simulink library "mbrt_lib_level1"  (R2023b)
settings: Solver=VariableStepAuto  StartTime=0.0  StopTime=10.0  RelTol=1e-3
values from neighbouring files (symbols this model uses):
  P_cpid_BehaviorPublish = uint64(12)    [i01_data.m]
  P_cpid_CameraStart = uint64(1)    [i01_data.m]
undefined symbols (not defined in the file or in its folder): cpseq, cpseq_SL_Info, cur_cpid, health, seqctr, time
libraries: ros2lib x4, mbrt_lib_level0 x2
settings Model: Creator=ftraenkle  LastModifiedBy=ftraenkle
settings SolverCC: AlgebraicLoopSolver=TrustRegion
settings OptimizationCC: ReuseModelBlockBuffer=off
settings DebuggingCC: UnconnectedInputMsg=warning  UnconnectedOutputMsg=warning  UnconnectedLineMsg=warning
settings ModelReferenceCC: EnableRefExpFcnMdlSchedulingChecks=on
settings RTWCC: DLArmComputeVersion=19.05

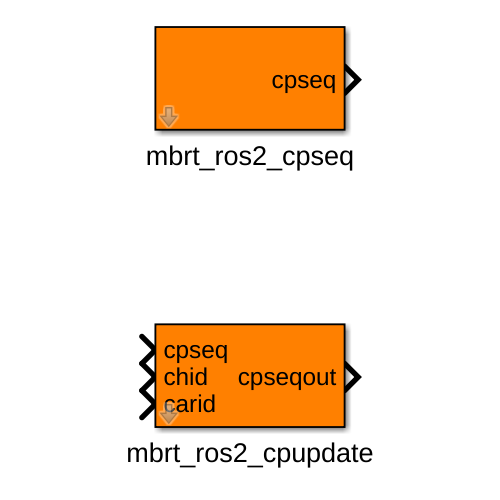
[thumbnail: Simulink's stored preview of the top-level diagram]
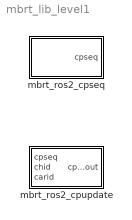
== system mbrt_lib_level1 ==
  mbrt_ros2_cpseq : Subsystem  mask{P_cur_cpid=P_cpid_CameraStart}
      mask prompts: P_cur_cpid "Current Checkpoint Id"
  mbrt_ros2_cpupdate : Subsystem  mask{P_cur_cpid=P_cpid_BehaviorPublish}
      mask prompts: P_cur_cpid "Current Checkpoint Id"

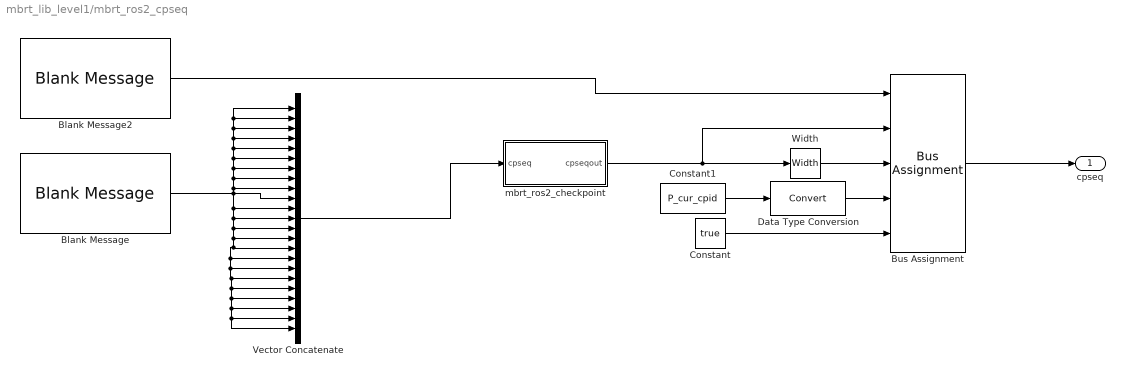
== system mbrt_lib_level1/mbrt_ros2_cpseq ==
  Blank Message : ros2lib/Blank Message  messageClass=Message  entityType=mbsafemsgs/Checkpoint  messageType=mbsafemsgs/Checkpoint  SampleTime=inf
  Blank Message2 : ros2lib/Blank Message  messageClass=Message  entityType=mbsafemsgs/CheckpointSequence  messageType=mbsafemsgs/CheckpointSequence  SampleTime=inf
  Bus Assignment : BusAssignment  AssignedSignals=cpseq,cpseq_SL_Info.CurrentLength,cur_cpid,health
  Constant : Constant  Value=true  OutDataTypeStr=boolean
  Constant1 : Constant  Value=P_cur_cpid
  Data Type Conversion : DataTypeConversion  SaturateOnIntegerOverflow=off  RndMeth=Floor
  Vector Concatenate : Concatenate  NumInputs=P_cp_cnt
  Width : Width  DataType=uint32
  mbrt_ros2_checkpoint : Subsystem
  cpseq : Outport
  wires:
  mbrt_ros2_checkpoint/1(cpseqout) -> Width/1, Bus Assignment/2
  Blank Message2/1 -> Bus Assignment/1
  Data Type Conversion/1 -> Bus Assignment/4
  Blank Message/1 -> Vector Concatenate/8, Vector Concatenate/7, Vector Concatenate/6, Vector Concatenate/5, Vector Concatenate/1, Vector Concatenate/2, Vector Concatenate/3, Vector Concatenate/4, Vector Concatenate/9, Vector Concatenate/10, Vector Concatenate/11, Vector Concatenate/12, Vector Concatenate/13, Vector Concatenate/14, Vector Concatenate/15, Vector Concatenate/17, Vector Concatenate/18, Vector Concatenate/19, Vector Concatenate/20, Vector Concatenate/21, Vector Concatenate/23, Vector Concatenate/22, Vector Concatenate/16
  Vector Concatenate/1 -> mbrt_ros2_checkpoint/1(cpseq)
  Width/1 -> Bus Assignment/3
  Bus Assignment/1 -> cpseq/1
  Constant1/1 -> Data Type Conversion/1
  Constant/1 -> Bus Assignment/5

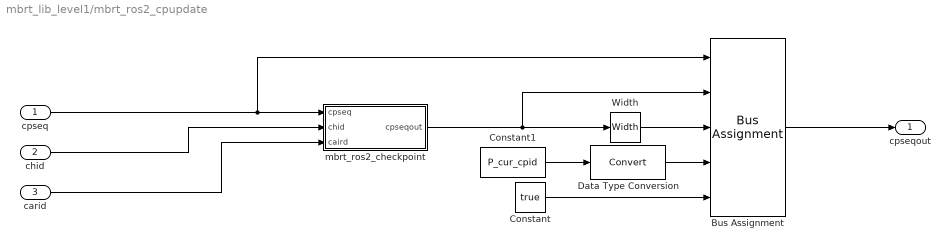
== system mbrt_lib_level1/mbrt_ros2_cpupdate ==
  cpseq : Inport
  chid : Inport  Port=2
  carid : Inport  Port=3
  Bus Assignment : BusAssignment  AssignedSignals=cpseq,cpseq_SL_Info.CurrentLength,cur_cpid,health
  Constant : Constant  Value=true  OutDataTypeStr=boolean
  Constant1 : Constant  Value=P_cur_cpid
  Data Type Conversion : DataTypeConversion  SaturateOnIntegerOverflow=off  RndMeth=Floor
  Width : Width  DataType=uint32
  mbrt_ros2_checkpoint : Subsystem
  cpseqout : Outport
  wires:
  carid/1 -> mbrt_ros2_checkpoint/3(caird)
  chid/1 -> mbrt_ros2_checkpoint/2(chid)
  Bus Assignment/1 -> cpseqout/1
  mbrt_ros2_checkpoint/1(cpseqout) -> Width/1, Bus Assignment/2
  Data Type Conversion/1 -> Bus Assignment/4
  Width/1 -> Bus Assignment/3
  cpseq/1 -> mbrt_ros2_checkpoint/1(cpseq), Bus Assignment/1
  Constant1/1 -> Data Type Conversion/1
  Constant/1 -> Bus Assignment/5

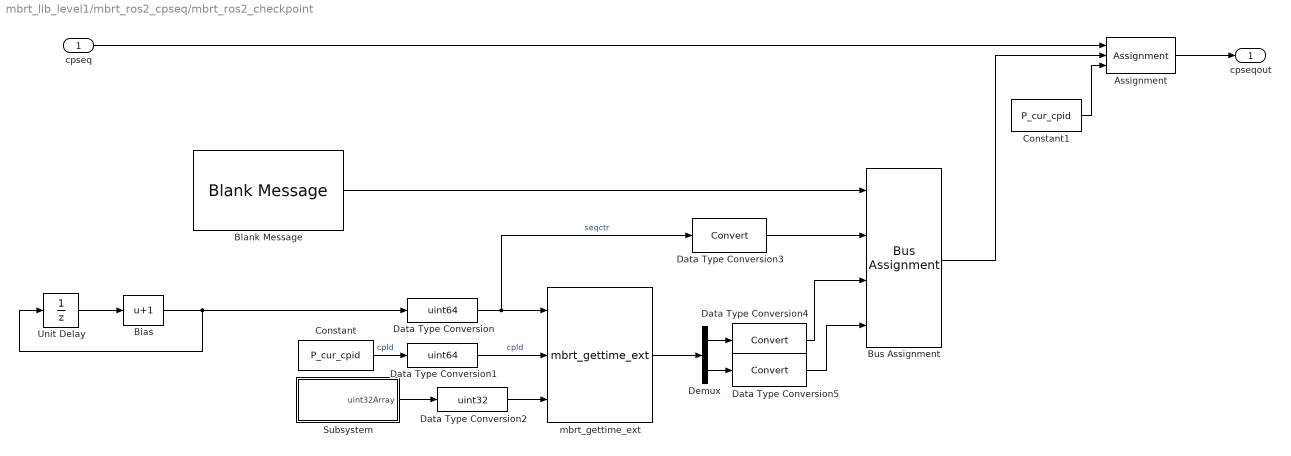
== system mbrt_lib_level1/mbrt_ros2_cpseq/mbrt_ros2_checkpoint ==
  cpseq : Inport
  Assignment : Assignment  IndexMode=Zero-based  DiagnosticForDimensions=Warning  IndexOptions=Index vector (port)  Indices=[1]  OutputSizes=1
  Bias : Bias  Bias=1  SaturateOnIntegerOverflow=off
  Blank Message : ros2lib/Blank Message  messageClass=Message  entityType=mbsafemsgs/Checkpoint  messageType=mbsafemsgs/Checkpoint  SampleTime=inf
  Bus Assignment : BusAssignment  AssignedSignals=seqctr,time.sec,time.nanosec
  Constant : Constant  Value=P_cur_cpid
  Constant1 : Constant  Value=P_cur_cpid
  Data Type Conversion : DataTypeConversion  OutDataTypeStr=uint64  SaturateOnIntegerOverflow=off  RndMeth=Floor
  Data Type Conversion1 : DataTypeConversion  OutDataTypeStr=uint64  SaturateOnIntegerOverflow=off  RndMeth=Floor
  Data Type Conversion2 : DataTypeConversion  OutDataTypeStr=uint32  SaturateOnIntegerOverflow=off  RndMeth=Floor
  Data Type Conversion3 : DataTypeConversion  SaturateOnIntegerOverflow=off  RndMeth=Floor
  Data Type Conversion4 : DataTypeConversion  SaturateOnIntegerOverflow=off  RndMeth=Floor
  Data Type Conversion5 : DataTypeConversion  SaturateOnIntegerOverflow=off  RndMeth=Floor
  Demux : Demux  Outputs=2
  Subsystem : Subsystem
  Unit Delay : UnitDelay  InitialCondition=uint64(0)  SampleTime=-1  HasFrameUpgradeWarning=on
  mbrt_gettime_ext : mbrt_lib_level0/mbrt_gettime_ext
  cpseqout : Outport
  wires:
  Constant1/1 -> Assignment/3
  cpseq/1 -> Assignment/1
  Assignment/1 -> cpseqout/1
  Bus Assignment/1 -> Assignment/2
  Data Type Conversion5/1 -> Bus Assignment/4
  Data Type Conversion4/1 -> Bus Assignment/3
  Data Type Conversion3/1 -> Bus Assignment/2
  Blank Message/1 -> Bus Assignment/1
  Data Type Conversion/1 -> mbrt_gettime_ext/1, Data Type Conversion3/1  "seqctr"
  Subsystem/1(uint32Array) -> Data Type Conversion2/1
  Demux/2 -> Data Type Conversion5/1
  Demux/1 -> Data Type Conversion4/1
  Unit Delay/1 -> Bias/1
  Data Type Conversion2/1 -> mbrt_gettime_ext/3
  Data Type Conversion1/1 -> mbrt_gettime_ext/2  "cpId"
  Constant/1 -> Data Type Conversion1/1  "cpId"
  Bias/1 -> Data Type Conversion/1, Unit Delay/1
  mbrt_gettime_ext/1 -> Demux/1

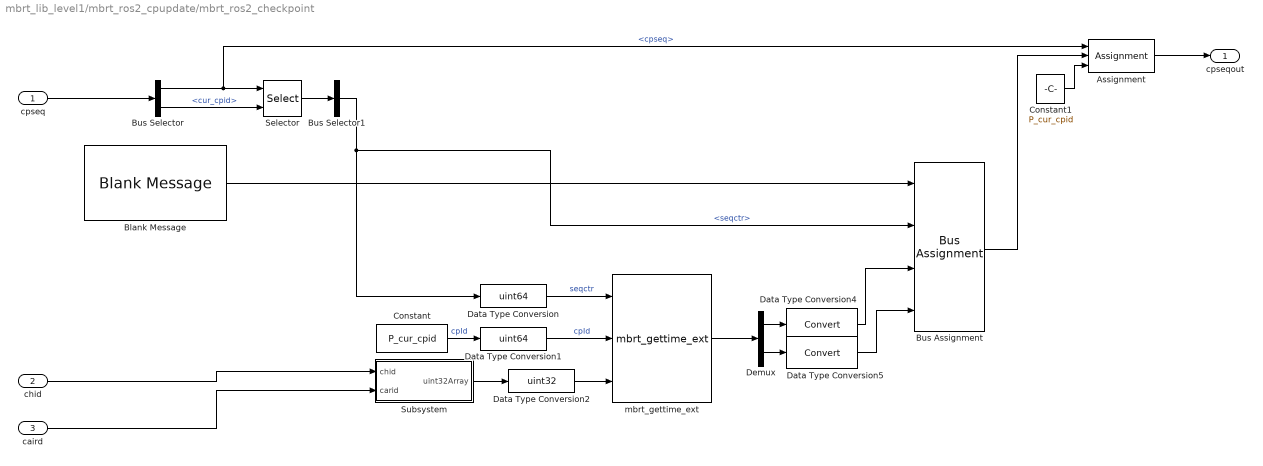
== system mbrt_lib_level1/mbrt_ros2_cpupdate/mbrt_ros2_checkpoint ==
  cpseq : Inport
  chid : Inport  Port=2
  caird : Inport  Port=3
  Assignment : Assignment  IndexMode=Zero-based  DiagnosticForDimensions=Warning  IndexOptions=Index vector (port)  Indices=[1]  OutputSizes=1
  Blank Message : ros2lib/Blank Message  messageClass=Message  entityType=mbsafemsgs/Checkpoint  messageType=mbsafemsgs/Checkpoint  SampleTime=inf
  Bus Assignment : BusAssignment  AssignedSignals=seqctr,time.sec,time.nanosec
  Bus Selector : BusSelector  OutputSignals=cpseq,cur_cpid
  Bus Selector1 : BusSelector  OutputSignals=seqctr
  Constant : Constant  Value=P_cur_cpid
  Constant1 : Constant  Value=P_cur_cpid
  Data Type Conversion : DataTypeConversion  OutDataTypeStr=uint64  SaturateOnIntegerOverflow=off  RndMeth=Floor
  Data Type Conversion1 : DataTypeConversion  OutDataTypeStr=uint64  SaturateOnIntegerOverflow=off  RndMeth=Floor
  Data Type Conversion2 : DataTypeConversion  OutDataTypeStr=uint32  SaturateOnIntegerOverflow=off  RndMeth=Floor
  Data Type Conversion4 : DataTypeConversion  SaturateOnIntegerOverflow=off  RndMeth=Floor
  Data Type Conversion5 : DataTypeConversion  SaturateOnIntegerOverflow=off  RndMeth=Floor
  Demux : Demux  Outputs=2
  Selector : Selector  IndexMode=Zero-based  InputPortWidth=P_cp_cnt  IndexOptions=Index vector (port)  Indices=[1 3]  OutputSizes=1
  Subsystem : Subsystem
  mbrt_gettime_ext : mbrt_lib_level0/mbrt_gettime_ext
  cpseqout : Outport
  wires:
  caird/1 -> Subsystem/2(carid)
  chid/1 -> Subsystem/1(chid)
  Constant1/1 -> Assignment/3
  Bus Selector1/1 -> Data Type Conversion/1, Bus Assignment/2  "<seqctr>"
  Selector/1 -> Bus Selector1/1
  Bus Selector/1 -> Selector/1, Assignment/1  "<cpseq>"
  Bus Selector/2 -> Selector/2  "<cur_cpid>"
  cpseq/1 -> Bus Selector/1
  Assignment/1 -> cpseqout/1
  Bus Assignment/1 -> Assignment/2
  Data Type Conversion5/1 -> Bus Assignment/4
  Data Type Conversion4/1 -> Bus Assignment/3
  Blank Message/1 -> Bus Assignment/1
  Data Type Conversion/1 -> mbrt_gettime_ext/1  "seqctr"
  Subsystem/1(uint32Array) -> Data Type Conversion2/1
  Demux/2 -> Data Type Conversion5/1
  Demux/1 -> Data Type Conversion4/1
  Data Type Conversion2/1 -> mbrt_gettime_ext/3
  Data Type Conversion1/1 -> mbrt_gettime_ext/2  "cpId"
  Constant/1 -> Data Type Conversion1/1  "cpId"
  mbrt_gettime_ext/1 -> Demux/1

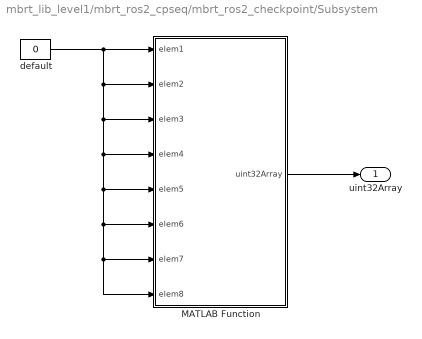
== system mbrt_lib_level1/mbrt_ros2_cpseq/mbrt_ros2_checkpoint/Subsystem ==
  MATLAB Function : MATLAB Function  TreatAsAtomicUnit=on
  default : Constant  Value=0  OutDataTypeStr=uint32
  uint32Array : Outport
  wires:
  default/1 -> MATLAB Function/8(elem8), MATLAB Function/7(elem7), MATLAB Function/6(elem6), MATLAB Function/5(elem5), MATLAB Function/4(elem4), MATLAB Function/3(elem3), MATLAB Function/2(elem2), MATLAB Function/1(elem1)
  MATLAB Function/1(uint32Array) -> uint32Array/1

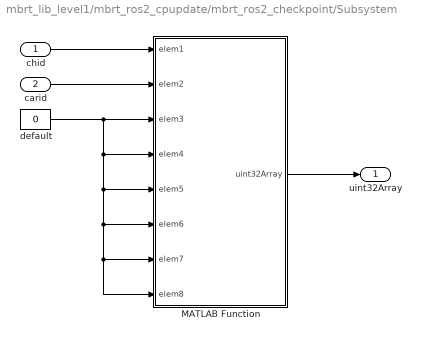
== system mbrt_lib_level1/mbrt_ros2_cpupdate/mbrt_ros2_checkpoint/Subsystem ==
  chid : Inport
  carid : Inport  Port=2
  MATLAB Function : MATLAB Function  TreatAsAtomicUnit=on
  default : Constant  Value=0  OutDataTypeStr=uint32
  uint32Array : Outport
  wires:
  carid/1 -> MATLAB Function/2(elem2)
  chid/1 -> MATLAB Function/1(elem1)
  MATLAB Function/1(uint32Array) -> uint32Array/1
  default/1 -> MATLAB Function/3(elem3), MATLAB Function/4(elem4), MATLAB Function/5(elem5), MATLAB Function/6(elem6), MATLAB Function/7(elem7), MATLAB Function/8(elem8)

== matlab function mbrt_lib_level1/mbrt_ros2_cpupdate/mbrt_ros2_checkpoint/Subsystem/MATLAB Function ==
  data: elem1 input; uint32Array output; elem2 input; elem3 input; elem4 input; elem5 input; elem6 input; elem7 input; elem8 input
function uint32Array = fcn(elem1, elem2, elem3, elem4, elem5, elem6, elem7, elem8)

uint32Array = [elem1, elem2, elem3, elem4, elem5, elem6, elem7, elem8;];

end

== matlab function mbrt_lib_level1/mbrt_ros2_cpseq/mbrt_ros2_checkpoint/Subsystem/MATLAB Function ==
  data: elem1 input; uint32Array output; elem2 input; elem3 input; elem4 input; elem5 input; elem6 input; elem7 input; elem8 input
function uint32Array = fcn(elem1, elem2, elem3, elem4, elem5, elem6, elem7, elem8)

uint32Array = [elem1, elem2, elem3, elem4, elem5, elem6, elem7, elem8;];
